simulink model "translationalkinematics"  (R2023a)
settings: Solver=ode45  StartTime=0.0  StopTime=1000.0  RelTol=1e-3
undefined symbols (not defined in the file): pitch, roll, x0, yaw
libraries: matrix_library x2
settings Model: Creator=prafulsigdel  LastModifiedBy=prafulsigdel

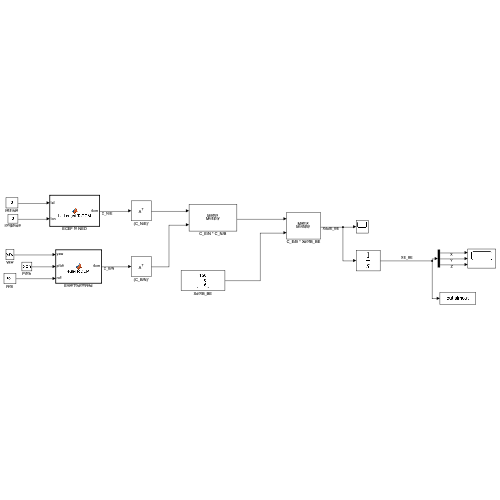
[thumbnail: Simulink's stored preview of the top-level diagram]
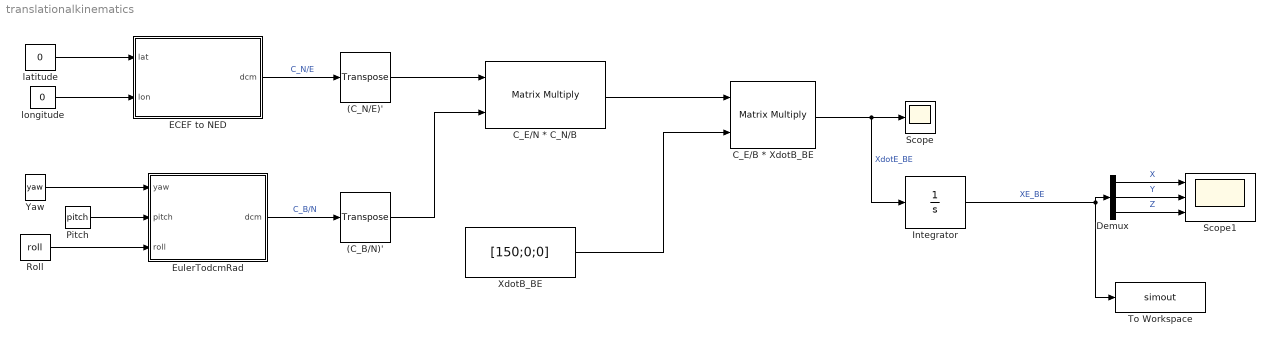
== system translationalkinematics ==
  (C_B/N)' : matrix_library/Transpose
  (C_N/E)' : matrix_library/Transpose
  C_E/B * XdotB_BE : Product  Multiplication=Matrix(*)
  C_E/N * C_N/B : Product  Multiplication=Matrix(*)
  Demux : Demux  Outputs=3
  ECEF to NED : MATLAB Function  TreatAsAtomicUnit=on
  EulerTodcmRad : MATLAB Function  TreatAsAtomicUnit=on
  Integrator : Integrator  InitialCondition=x0
  Pitch : Constant  Value=pitch
  Roll : Constant  Value=roll
  Scope : Scope
  Scope1 : Scope  NumInputPorts=3
  To Workspace : ToWorkspace  VariableName=simout  SaveFormat=Timeseries  SampleTime=-1
  XdotB_BE : Constant  Value=[150;0;0]  VectorParams1D=off
  Yaw : Constant  Value=yaw
  latitude : Constant  Value=0
  longitude : Constant  Value=0
  wires:
  Yaw/1 -> EulerTodcmRad/1(yaw)
  Pitch/1 -> EulerTodcmRad/2(pitch)
  Roll/1 -> EulerTodcmRad/3(roll)
  EulerTodcmRad/1(dcm) -> (C_B/N)'/1  "C_B/N"
  (C_B/N)'/1 -> C_E/N * C_N/B/2
  ECEF to NED/1(dcm) -> (C_N/E)'/1  "C_N/E"
  (C_N/E)'/1 -> C_E/N * C_N/B/1
  latitude/1 -> ECEF to NED/1(lat)
  longitude/1 -> ECEF to NED/2(lon)
  C_E/B * XdotB_BE/1 -> Integrator/1, Scope/1  "XdotE_BE"
  XdotB_BE/1 -> C_E/B * XdotB_BE/2
  C_E/N * C_N/B/1 -> C_E/B * XdotB_BE/1
  Integrator/1 -> Demux/1, To Workspace/1  "XE_BE"
  Demux/3 -> Scope1/3  "Z"
  Demux/1 -> Scope1/1  "X"
  Demux/2 -> Scope1/2  "Y"

== matlab function translationalkinematics/EulerTodcmRad ==
  data: yaw input; dcm output; pitch input; roll input
function dcm = eulerToDCM(yaw, pitch, roll)
% Convert euler angles to DCM angles in Radians.
C_Y = [cos(yaw) -sin(yaw) 0; sin(yaw) cos(yaw) 0;0 0 1];
C_P = [cos(pitch) 0 sin(pitch); 0 1 0; -sin(pitch) 0 cos(pitch)];
C_R = [1 0 0; 0 cos(roll) -sin(roll); 0 sin(roll) cos(roll)];

% Convert DCM
dcm = C_R * C_P * C_Y;

end

== matlab function translationalkinematics/ECEF to NED ==
  data: lat input; dcm output; lon input
function dcm = LatLongAttToDCM(lat, lon)
% Convert euler angles to DCM
C_NE = [0 0 1; 0 1 0; -1 0 0];
C_NdN = [cos(lat) 0 sin(lat); 0 1 0; -sin(lat) 0 cos(lat)];
C_NNd = [1 0 0; 0 cos(lon) -sin(lon); 0 sin(lon) cos(lon)];

% Convert DCM
dcm = C_NNd * C_NdN * C_NE;

end
